simulink model "mobil_transporter"  (R2012b)
settings: Solver=FixedStepDiscrete  StartTime=0.0  StopTime=10.0  RelTol=1e-3
libraries: commutil2 x12, c2833xlib x8, c280xlib x6, idelinklib_tgtpref x2, simulink x1, idelinklib_ticcs x1
(part 2 of 2)

== stateflow chart mobil_transporter/Modul Positionswerte Sampletime = 0.01 s/Chart8 ==
  state wert_erkannt
    entry:
    values_out1[0] = in_data[0];
    values_out1[1] = in_data[1];
    values_out1[2] = in_data[2];
    values_out1[3] = in_data[3];
    values_out1[4] = in_data[4];
    values_out1[5] = in_data[5];
    values_out1[6] = in_data[6];
    values_out1[7] = in_data[7];
    values_out1[8] = in_data[8];
    values_out1[9] = in_data[9];
    values_out1[10] = in_data[10];
    values_out1[11] = in_data[11];
    values_out1[12] = in_data[12];
    values_out1[13] = in_data[13];
    values_out1[14] = in_data[14];
    values_out1[15] = in_data[15];
    values_out1[16] = in_data[16];
    values_out1[17] = in_data[17];
    values_out1[18] = in_data[18];
    values_out1[19] = in_data[19];
  state init
    values_out1[0] = 0;
    values_out1[1] = 0;
    values_out1[2] = 0;
    values_out1[3] = 0;
    values_out1[4] = 0;
    values_out1[5] = 0;
    values_out1[6] = 0;
    values_out1[7] = 0;
    values_out1[8] = 0;
    values_out1[9] = 0;
    values_out1[10] = 0;
    values_out1[11] = 0;
    values_out1[12] = 0;
    values_out1[13] = 0;
    values_out1[14] = 0;
    values_out1[15] = 0;
    values_out1[16] = 0;
    values_out1[17] = 0;
    values_out1[18] = 0;
    values_out1[19] = 0;
  state Anfang_found_Schritt_uebertragen_weglassen_performance
    x_found = x_found +1;
  state x5_valid_data_found1
    valid_values1 = values_out1[search+1];
    valid_values2 = values_out1[search+2];
    valid_values3 = values_out1[search+3];
    valid_values4 = values_out1[search+4];
    valid_values5 = values_out1[search+5];
    valid_values6 = values_out1[search+6];
    valid_values7 = values_out1[search+7];
    valid_values8 = values_out1[search+8];
    zaehler = zaehler +1;
  state wert_erkannt2
    entry:
    search = 0;
    counter = counter + 1;
  state x1_search1
    search = search + 1;
  x5_valid_data_found1 -> wert_erkannt
  (default) -> init
  x1_search1 -> wert_erkannt [order 3]
  init -> wert_erkannt
  Anfang_found_Schritt_uebertragen_weglassen_performance -> x5_valid_data_found1 [order 1] : [((values_out1[search]+values_out1[search+1]+values_out1[search+2]+values_out1[search+3]+values_out1[search+4]+values_out1[search+5]+values_out1[search+6]+values_out1[search+7]+values_out1[search+8])) == values_out1[search+9]]
  Anfang_found_Schritt_uebertragen_weglassen_performance -> x5_valid_data_found1 [order 2] : [((values_out1[search]+values_out1[search+1]+values_out1[search+2]+values_out1[search+3]+values_out1[search+4]+values_out1[search+5]+values_out1[search+6]+values_out1[search+7]+values_out1[search+8])-(256)) == values_out1[search+9]]
  wert_erkannt -> wert_erkannt2
  Anfang_found_Schritt_uebertragen_weglassen_performance -> x5_valid_data_found1 [order 3] : [((values_out1[search]+values_out1[search+1]+values_out1[search+2]+values_out1[search+3]+values_out1[search+4]+values_out1[search+5]+values_out1[search+6]+values_out1[search+7]+values_out1[search+8])-(512)) == values_out1[search+9]]
  Anfang_found_Schritt_uebertragen_weglassen_performance -> x5_valid_data_found1 [order 7] : [((values_out1[search]+values_out1[search+1]+values_out1[search+2]+values_out1[search+3]+values_out1[search+4]+values_out1[search+5]+values_out1[search+6]+values_out1[search+7]+values_out1[search+8])-(768)) == values_out1[search+9]]
  Anfang_found_Schritt_uebertragen_weglassen_performance -> x5_valid_data_found1 [order 6] : [((values_out1[search]+values_out1[search+1]+values_out1[search+2]+values_out1[search+3]+values_out1[search+4]+values_out1[search+5]+values_out1[search+6]+values_out1[search+7]+values_out1[search+8])-(1024)) == values_out1[search+9]]
  Anfang_found_Schritt_uebertragen_weglassen_performance -> x5_valid_data_found1 [order 5] : [((values_out1[search]+values_out1[search+1]+values_out1[search+2]+values_out1[search+3]+values_out1[search+4]+values_out1[search+5]+values_out1[search+6]+values_out1[search+7]+values_out1[search+8])-(1280)) == values_out1[search+9]]
  Anfang_found_Schritt_uebertragen_weglassen_performance -> x5_valid_data_found1 [order 4] : [((values_out1[search]+values_out1[search+1]+values_out1[search+2]+values_out1[search+3]+values_out1[search+4]+values_out1[search+5]+values_out1[search+6]+values_out1[search+7]+values_out1[search+8])-(1536)) == values_out1[search+9]]
  Anfang_found_Schritt_uebertragen_weglassen_performance -> x5_valid_data_found1 [order 8] : [((values_out1[search]+values_out1[search+1]+values_out1[search+2]+values_out1[search+3]+values_out1[search+4]+values_out1[search+5]+values_out1[search+6]+values_out1[search+7]+values_out1[search+8])-(1792)) == values_out1[search+9]]
  Anfang_found_Schritt_uebertragen_weglassen_performance -> x5_valid_data_found1 [order 10] : [((values_out1[search]+values_out1[search+1]+values_out1[search+2]+values_out1[search+3]+values_out1[search+4]+values_out1[search+5]+values_out1[search+6]+values_out1[search+7]+values_out1[search+8])-(2048)) == values_out1[search+9]]
  Anfang_found_Schritt_uebertragen_weglassen_performance -> x1_search1 [order 9]
  wert_erkannt2 -> Anfang_found_Schritt_uebertragen_weglassen_performance [order 1] : [values_out1[search] == 88]
  x1_search1 -> Anfang_found_Schritt_uebertragen_weglassen_performance [order 1] : [values_out1[search] == 88]
  wert_erkannt2 -> x1_search1 [order 2]
  x1_search1 -> x1_search1 [order 2] : [search < 19]
  data: in_data input size=20; values_out1 local int16 size=20; zaehler local int32 =0; search local int16; valid_values1 output int16 size=1; valid_values2 output int16 size=1; valid_values3 output int16 size=1; valid_values4 output int16 size=1; valid_values5 output int16 size=1; valid_values6 output int16 size=1; valid_values7 output int16 size=1; valid_values8 output int16 size=1; counter local int32 =0; x_found local int32 =0

== matlab function mobil_transporter/Navigation/Winkel Bereich Bestimmen damit die Richtung der Motoren bestimmet und den entsprechden Regler verwendet werden/WinkelVergleich ==
  settings: updateMethod=DISCRETE  sampleTime=0.01
  data: u input; W output
function W = fcn( u)
if 15 <= u && u <= 180 || -345 <= u && u <= -180
    %%Linksabbiegen
    W = 1;
elseif -180 < u && u < -15 || 180 < u && u < 345
    %%Rechtsabbiegen
    W = 2;
else
    %%Gerade Fahren
    W = 0;
   
end

== matlab function mobil_transporter/Modul Positionswerte Sampletime = 0.01 s/I2C Reset (behebt Stabilitätsprobleme der I2C-Verbindung)/I2C Reinitialisierung/I2C Reinitialisierung ==
function fcn()
%#codegen

coder.ceval( 'init_i2c' );

== matlab function mobil_transporter/Modul Positionswerte Sampletime = 0.01 s/I2C Reset (behebt Stabilitätsprobleme der I2C-Verbindung)/I2C Reset/I2C Reset ==
function fcn()
%#codegen

coder.ceval( 'reset_i2c' );
